simulink model "Prosthetic_Leg"  (R2013a)
settings: Solver=ode15s  StartTime=0.0  StopTime=10  MaxStep=.01  RelTol=1e-3
libraries: simulink x1
settings Model: Creator=jander13  LastModifiedBy=rlwood08

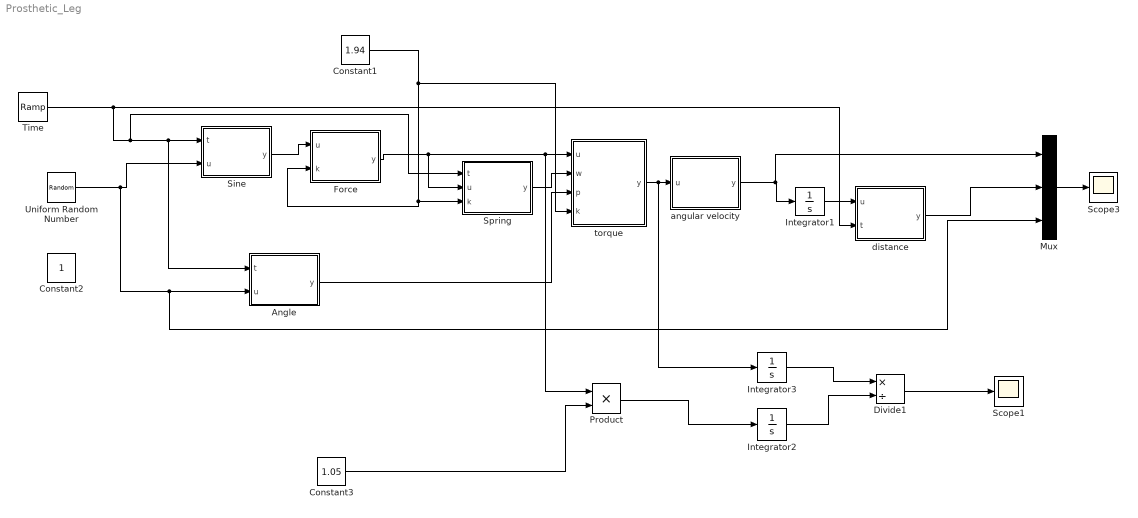
== system Prosthetic_Leg ==
  Angle : MATLAB Function  TreatAsAtomicUnit=on
  Constant1 : Constant  Value=1.94
  Constant2 : Constant
  Constant3 : Constant  Value=1.05
  Divide1 : Product  Inputs=*/
  Force : MATLAB Function  TreatAsAtomicUnit=on
  Integrator1 : Integrator
  Integrator2 : Integrator
  Integrator3 : Integrator
  Mux : Mux  Inputs=3
  Product : Product
  Scope1 : Scope
      settings: YMin=-1  YMax=17
  Scope3 : Scope
      settings: ShowLegends=on  YMin=-1  YMax=17  SaveName=ScopeData3
  Sine : MATLAB Function  TreatAsAtomicUnit=on
  Spring : MATLAB Function  TreatAsAtomicUnit=on
  Time : simulink/Sources/Ramp  slope=1  start=0  X0=.01
  Uniform Random Number : UniformRandomNumber  Minimum=0  Maximum=2  Seed=1  SampleTime=2
  angular velocity : MATLAB Function  TreatAsAtomicUnit=on
  distance : MATLAB Function  TreatAsAtomicUnit=on
  "torque " : MATLAB Function  TreatAsAtomicUnit=on
  wires:
  Sine/1(y) -> Force/1(u)
  "torque "/1(y) -> Integrator3/1, angular velocity/1(u)
  Force/1(y) -> Spring/2(u), Product/1, "torque "/1(u)
  Time/1 -> distance/2(t), Spring/1(t), Angle/1(t), Sine/1(t)
  Mux/1 -> Scope3/1
  Angle/1(y) -> "torque "/3(p)
  Integrator1/1 -> distance/1(u)
  angular velocity/1(y) -> Mux/1, Integrator1/1
  Constant1/1 -> "torque "/4(k), Force/2(k), Spring/3(k)
  distance/1(y) -> Mux/2
  Uniform Random Number/1 -> Mux/3, Angle/2(u), Sine/2(u)
  Spring/1(y) -> "torque "/2(w)
  Integrator2/1 -> Divide1/2
  Integrator3/1 -> Divide1/1
  Divide1/1 -> Scope1/1
  Product/1 -> Integrator2/1
  Constant3/1 -> Product/2

== matlab function Prosthetic_Leg/Force ==
  data: u input; y output; k input
function y = fcn(u,k)

   z=u;
    
    if z>0
        z=k*1.05+9.81*2.7*3/2;
    end
    
y =z ;

== matlab function Prosthetic_Leg/Sine ==
  data: t input; u input; y output
function y = fcn(t,u)

    z=u*sin(2*pi()*t);
    x=u*sin(pi()*t);
        
    if z<0 | x<0
        z=0
    end
   
y =z ;

== matlab function Prosthetic_Leg/torque  ==
  data: u input; y output; w input; p input; k input
function y = fcn(u,w,p,k)

L=.8;
m=2.7;
g=9.81;


z=-u*L/3*sin(p)+k*w*L/3*sin(p)+m*g*L/2*sin(p);
    
   
y =z ;

== matlab function Prosthetic_Leg/Spring ==
  data: t input; u input; y output; k input
function y = fcn(t,u,k)

l=u;
g = k;
z= 0;
if l > 0
    z = 1/g*(1-cos(g*t));
end

y = z;

== matlab function Prosthetic_Leg/angular velocity ==
  data: u input; y output
function y = fcn(u)

c = u;
m = 2.7;
L = .8;
   
y = 3*c/(m*L^2);

== matlab function Prosthetic_Leg/Angle ==
  data: t input; u input; y output
function y = fcn(t,u)

    z=pi()/4*u*sin(pi()*t);
    if z<0 
        z=0;
    end    
    
    y = z;

== matlab function Prosthetic_Leg/distance ==
  data: u input; y output; t input
function y = fcn(u,t)
c=u;

y = c/2;
